simulink model "prob4"  (R2020b)
settings: Solver=VariableStepAuto  StartTime=0.0  StopTime=10  RelTol=1e-3
values from neighbouring files (symbols this model uses):
  b = 3.5077E-6    [DATA1A.sldd]
  J = 3.2284E-6    [DATA1A.sldd]
  kd = 0.489767517465838    [DATA1A.sldd]
  Ke = 0.0274    [DATA1A.sldd]
  ki = 4810.14360766501    [DATA1A.sldd]
  kp = 97.1186920193705    [DATA1A.sldd]
  Kt = 0.0274    [DATA1A.sldd]
  L = 2.75E-6    [DATA1A.sldd]
  n = 119827.875340723    [DATA1A.sldd]
  R = 4.0    [DATA1A.sldd]
settings Model: DataDictionary=DATA1A.sldd  Creator=Hp  LastModifiedBy=Hp

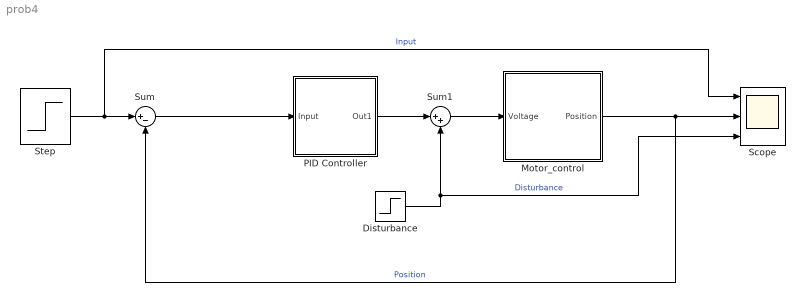
== system prob4 ==
  Disturbance : Step  Time=0.06  SampleTime=0
  Motor_control : Subsystem
  PID Controller : Subsystem  TreatAsAtomicUnit=on
  Scope : Scope  NumInputPorts=3
  Step : Step  Time=0  After=10  SampleTime=0
  Sum : Sum  Inputs=|+-
  Sum1 : Sum  Inputs=|++
  wires:
  Motor_control/1(Position) -> Sum/2, Scope/2  "Position"
  Disturbance/1 -> Sum1/2, Scope/3  "Disturbance"
  Step/1 -> Scope/1, Sum/1  "Input"
  Sum1/1 -> Motor_control/1(Voltage)
  PID Controller/1(Out1) -> Sum1/1
  Sum/1 -> PID Controller/1(Input)

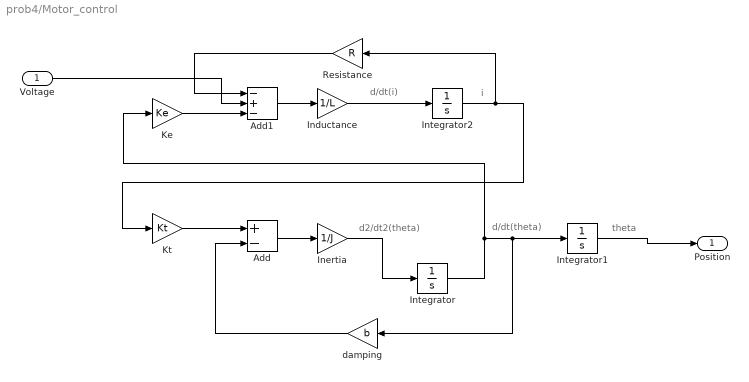
== system prob4/Motor_control ==
  note: i
  note: d/dt(i)
  note: theta
  note: d/dt(theta)
  note: d2/dt2(theta)
  Voltage : Inport
  Add : Sum  Inputs=+-
  Add1 : Sum  Inputs=-+-
  Inductance : Gain  Gain=1/L
  Inertia : Gain  Gain=1/J
  Integrator : Integrator
  Integrator1 : Integrator
  Integrator2 : Integrator
  Ke : Gain  Gain=Ke
  Kt : Gain  Gain=Kt
  Resistance : Gain  Gain=R
  damping : Gain  Gain=b
  Position : Outport
  wires:
  Add/1 -> Inertia/1
  Inductance/1 -> Integrator2/1
  Add1/1 -> Inductance/1
  Ke/1 -> Add1/3
  Integrator/1 -> Ke/1, damping/1, Integrator1/1
  damping/1 -> Add/2
  Inertia/1 -> Integrator/1
  Kt/1 -> Add/1
  Integrator2/1 -> Resistance/1, Kt/1
  Resistance/1 -> Add1/1
  Voltage/1 -> Add1/2
  Integrator1/1 -> Position/1

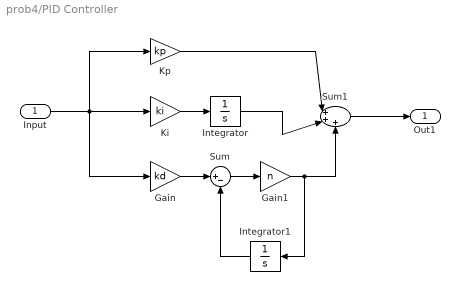
== system prob4/PID Controller ==
  Input : Inport
  Gain : Gain  Gain=kd
  Gain1 : Gain  Gain=n
  Integrator : Integrator
  Integrator1 : Integrator
  Ki : Gain  Gain=ki
  Kp : Gain  Gain=kp
  Sum : Sum  Inputs=|+-
  Sum1 : Sum  Inputs=|+++
  Out1 : Outport
  wires:
  Input/1 -> Gain/1, Ki/1, Kp/1
  Kp/1 -> Sum1/1
  Ki/1 -> Integrator/1
  Integrator/1 -> Sum1/2
  Gain/1 -> Sum/1
  Sum/1 -> Gain1/1
  Gain1/1 -> Integrator1/1, Sum1/3
  Integrator1/1 -> Sum/2
  Sum1/1 -> Out1/1
